simulink model "models"  (R2018a)
settings: Solver=VariableStepAuto  StartTime=0.0  StopTime=60  MaxStep=1e-3  RelTol=1e-3
values from neighbouring files (symbols this model uses):
  Droop_1 = 0.05    [ini_models.m]
  Droop_3 = 0.05    [ini_models.m]
  Kigov_1 = 2.0    (= 2)    [ini_models.m]
  Kigov_3 = 2.0    (= 2)    [ini_models.m]
  Kimw_1 = 0.01    [ini_models.m]
  Kimw_3 = 0.0    (= 0)    [ini_models.m]
  Kpgov_1 = 10.0    (= 10)    [ini_models.m]
  Kpgov_3 = 10.0    (= 10)    [ini_models.m]
  params = [T_1,T_2]    [ini_models.m]
  params_gov1 = [T_c_1,T_b_1,Kpgov_1,Kigov_1,Droop_1,Kimw_1]    [ini_models.m]
  params_pss = [T_w,T_pss_1,T_pss_2]    [ini_models.m]
  T_1 = 0.2    [ini_models.m]
  T_2 = 0.1    [ini_models.m]
  T_b_1 = 10.0    (= 10)    [ini_models.m]
  T_b_3 = 10.0    (= 10)    [ini_models.m]
  T_c_1 = 2.0    (= 2)    [ini_models.m]
  T_c_3 = 2.0    (= 2)    [ini_models.m]
  T_pss_1 = 0.61204417    [ini_models.m]
  T_pss_2 = 0.01695186    [ini_models.m]
  T_w = 5.0    (= 5)    [ini_models.m]
settings Model: Creator=jmmau  LastModifiedBy=jmmau

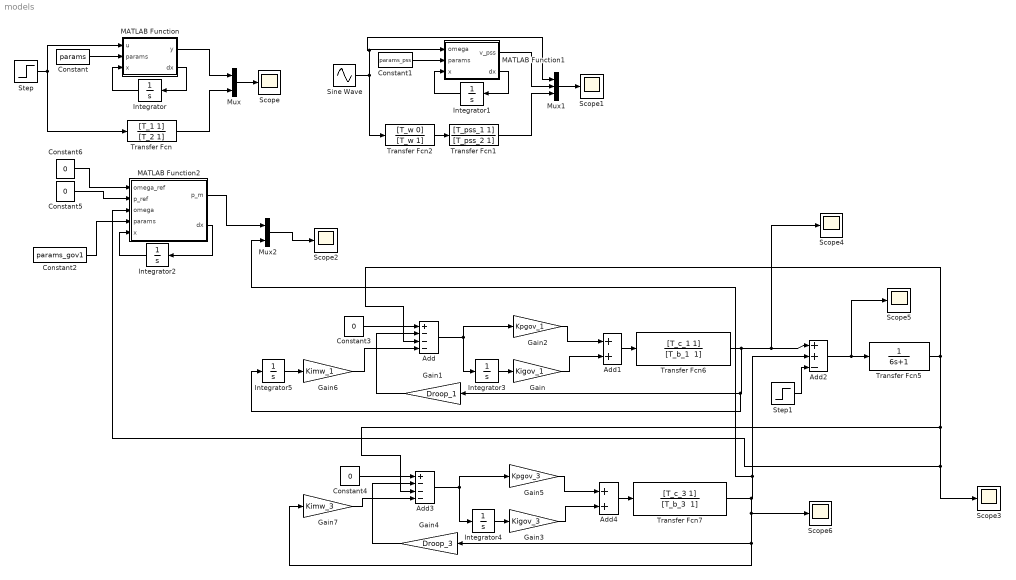
== system models ==
  Add : Sum  Inputs=+---
  Add1 : Sum
  Add2 : Sum  Inputs=++-
  Add3 : Sum  Inputs=+---
  Add4 : Sum
  Constant : Constant  Value=params
  Constant1 : Constant  Value=params_pss
  Constant2 : Constant  Value=params_gov1
  Constant{3..6} (4 alike) : Constant  Value=0
  Gain : Gain  Gain=Kigov_1
  Gain1 : Gain  Gain=Droop_1
  Gain2 : Gain  Gain=Kpgov_1
  Gain3 : Gain  Gain=Kigov_3
  Gain4 : Gain  Gain=Droop_3
  Gain5 : Gain  Gain=Kpgov_3
  Gain6 : Gain  Gain=Kimw_1
  Gain7 : Gain  Gain=Kimw_3
  Integrator{,3..5} (4 alike) : Integrator
  Integrator1 : Integrator  InitialCondition=[0,0]
  Integrator2 : Integrator  InitialCondition=[0,0,0,0]
  MATLAB Function : MATLAB Function  TreatAsAtomicUnit=on
  MATLAB Function1 : MATLAB Function  TreatAsAtomicUnit=on
  MATLAB Function2 : MATLAB Function  TreatAsAtomicUnit=on
  Mux : Mux  Inputs=2
  Mux1 : Mux  Inputs=3
  Mux2 : Mux  Inputs=2
  Scope{,1..6} (7 alike) : Scope
  Sine Wave : Sin  Frequency=9.817477042468102  SampleTime=0
  Step : Step  SampleTime=0
  Step1 : Step  SampleTime=0
  Transfer Fcn : TransferFcn  Numerator=[T_1 1]  Denominator=[T_2 1]
  Transfer Fcn1 : TransferFcn  Numerator=[T_pss_1 1]  Denominator=[T_pss_2 1]
  Transfer Fcn2 : TransferFcn  Numerator=[T_w 0]  Denominator=[T_w 1]
  Transfer Fcn5 : TransferFcn  Denominator="[6  1]"
  Transfer Fcn6 : TransferFcn  Numerator=[T_c_1 1]  Denominator="[T_b_1  1]"
  Transfer Fcn7 : TransferFcn  Numerator=[T_c_3 1]  Denominator="[T_b_3  1]"
  wires:
  MATLAB Function/2(dx) -> Integrator/1
  Integrator/1 -> MATLAB Function/3(x)
  Constant/1 -> MATLAB Function/2(params)
  Step/1 -> Transfer Fcn/1, MATLAB Function/1(u)
  MATLAB Function/1(y) -> Mux/1
  Transfer Fcn/1 -> Mux/2
  Mux/1 -> Scope/1
  MATLAB Function1/2(dx) -> Integrator1/1
  Sine Wave/1 -> Transfer Fcn2/1, Mux1/1, MATLAB Function1/1(omega)
  Integrator1/1 -> MATLAB Function1/3(x)
  Mux1/1 -> Scope1/1
  Constant1/1 -> MATLAB Function1/2(params)
  Transfer Fcn2/1 -> Transfer Fcn1/1
  MATLAB Function1/1(v_pss) -> Mux1/2
  Transfer Fcn1/1 -> Mux1/3
  Mux2/1 -> Scope2/1
  MATLAB Function2/2(dx) -> Integrator2/1
  Integrator2/1 -> MATLAB Function2/5(x)
  Constant2/1 -> MATLAB Function2/4(params)
  Constant3/1 -> Add/1
  Integrator3/1 -> Gain/1
  Gain/1 -> Add1/2
  Add1/1 -> Transfer Fcn6/1
  Gain2/1 -> Add1/1
  Add/1 -> Integrator3/1, Gain2/1
  Gain1/1 -> Add/2
  Add2/1 -> Scope5/1, Transfer Fcn5/1
  Transfer Fcn6/1 -> Integrator5/1, Gain1/1, Scope4/1, Add2/1
  Gain5/1 -> Add4/1
  Add3/1 -> Integrator4/1, Gain5/1
  Gain3/1 -> Add4/2
  Constant4/1 -> Add3/1
  Transfer Fcn5/1 -> Add3/3, MATLAB Function2/3(omega), Scope3/1, Add/3
  Add4/1 -> Transfer Fcn7/1
  Integrator4/1 -> Gain3/1
  Gain4/1 -> Add3/2
  Step1/1 -> Add2/3
  Transfer Fcn7/1 -> Scope6/1, Gain7/1, Gain4/1, Mux2/2, Add2/2
  Integrator5/1 -> Gain6/1
  Gain6/1 -> Add/4
  Gain7/1 -> Add3/4
  Constant5/1 -> MATLAB Function2/2(p_ref)
  Constant6/1 -> MATLAB Function2/1(omega_ref)
  MATLAB Function2/1(p_m) -> Mux2/1

== matlab function models/MATLAB Function1 ==
  data: omega input; params input; v_pss output; x input; dx output
function [v_pss,dx] = fcn(omega,params,x)

T_w = params(1);
T_pss_1 = params(2);
T_pss_2 = params(3);

x_pss =x(1);
x_w =x(2);

omega_w = omega - x_w;

dx_pss = (omega_w - x_pss)/T_pss_2;
dx_w =  (omega - x_w)/T_w;

v_pss = x_pss + T_pss_1/T_pss_2*(omega_w - x_pss);

dx = [dx_pss,dx_w];

% (T_1*s+1)/(T_2*s+1) = 1/(T_2*s+1) + (T_1*s)/(T_2*s+1)
% (T_1*s)/(T_2*s+1) = 1/(T_2*s+1) * T_1*s
% y = x_lead + T_1/T_2*(u - x_lead)

== matlab function models/MATLAB Function ==
  data: u input; params input; y output; x input; dx output
function [y,dx] = fcn(u,params,x)

T_1 = params(1);
T_2 = params(2);

x_lead = x;

dx_lead = (u - x_lead)/T_2;

y = x_lead + T_1/T_2*(u - x_lead);

dx = [dx_lead];

% (T_1*s+1)/(T_2*s+1) = 1/(T_2*s+1) + (T_1*s)/(T_2*s+1)
% (T_1*s)/(T_2*s+1) = 1/(T_2*s+1) * T_1*s
% y = x_lead + T_1/T_2*(u - x_lead)

== matlab function models/MATLAB Function2 ==
  data: omega_ref input; p_ref input; omega input; params input; p_m output; x input; dx output
function [p_m,dx] = fcn(omega_ref,p_ref,omega,params,x)

T_c = params(1);
T_b = params(2);
Kpgov = params(3);
Kigov = params(4);
Droop = params(5);
Kimw = params(6);

xi_gov =x(1);
xi_mw =x(2);
x_gov =x(3);
p_m_meas = x(4);


omega_droop = Droop*p_m_meas;
p_gov = Kpgov*(omega_ref - omega - omega_droop - Kimw*xi_mw) + Kigov*xi_gov;
p_m = x_gov + T_c/T_b*(p_gov - x_gov);

dxi_gov =  omega_ref - omega - omega_droop - Kimw*xi_mw;
dxi_mw = p_ref - p_m;
dx_gov = (p_gov - x_gov)/T_b;
dp_m_meas = 1/0.1*(p_m - p_m_meas);

dx = [dxi_gov,dxi_mw,dx_gov,dp_m_meas];

% (T_1*s+1)/(T_2*s+1) = 1/(T_2*s+1) + (T_1*s)/(T_2*s+1)
% (T_1*s)/(T_2*s+1) = 1/(T_2*s+1) * T_1*s
% y = x_lead + T_1/T_2*(u - x_lead)
